simulink model "Experience"  (R2025b)
settings: Solver=ode1  StartTime=0.0  StopTime=inf  FixedStep=0.005  RelTol=1e-3  EnableMultiTasking=on
values from neighbouring files (symbols this model uses):
  A = model.a    [param_control.m]
  B = model.b    [param_control.m]
  C = model.c    [param_control.m]
  H = 1/ (C_cmd*((eye(4) - A + B*K)\B))    [param_control.m]
  K = place(A, B, z_p)    [param_control.m]
  L = place(A',C', z_po)'    [param_control.m]
  nx = 4    [ident_model.m]    (also in param_control.m)
undefined symbols (not defined in the file or in its folder): Ka
libraries: arduinolib x1
settings Model: SimulationMode=external  ExtModeTrigDuration=2  Creator=Alex  LastModifiedBy=victor
settings SolverCC: AlgebraicLoopSolver=TrustRegion
settings DataIOCC: SaveFormat=StructureWithTime  ReturnWorkspaceOutputs=off
settings OptimizationCC: DefaultUnderspecifiedDataType=single  ReuseModelBlockBuffer=off  PassReuseOutputArgsAs=Individual arguments  MaxStackSize=64  EfficientTunableParamExpr=on
settings DebuggingCC: ParameterPrecisionLossMsg=none  ParameterTunabilityLossMsg=error  UnconnectedInputMsg=warning  UnconnectedOutputMsg=warning  UnconnectedLineMsg=warning  ArithmeticOperatorsInVariantConditions=warning
settings HardwareCC: ProdBitPerInt=16.0  ProdBitPerPointer=16.0  ProdBitPerSizeT=16.0  ProdBitPerPtrDiffT=16.0  ProdLargestAtomicFloat=None  ProdWordSize=8.0  ProdHWDeviceType=Atmel->AVR
settings ModelReferenceCC: EnableRefExpFcnMdlSchedulingChecks=on
settings SFSimCC: SimUseLocalCustomCode=off  MATLABDynamicMemAlloc=off  CustomCodeUndefinedFunction=UseInterfaceOnly
settings RTWCC: SystemTargetFile=ert.tlc  HardwareBoard=Arduino Mega 2560  TemplateMakefile=ert_default_tmf  RTWUseLocalCustomCode=off  Toolchain=Arduino AVR  BuildConfiguration=Faster Runs  IncludeHyperlinkInReport=on  GPUComputeCapability=3.5  DLArmComputeVersion=19.05  Description=Embedded Coder
settings CodeAppCC: ForceParamTrailComments=on  IgnoreCustomStorageClasses=off  OperatorAnnotations=on  SimulinkDataObjDesc=on  SFDataObjDesc=on  InsertBlockDesc=on
settings ERTTargetCC: ExtModeTransport=3.0  ExtModeStaticAlloc=on  ExtModeStaticAllocSize=1000.0  ExtModeMexFile=ext_xcp  ExtModeIntrfLevel=Level2 - Open  InlinedParameterPlacement=Hierarchical  DynamicArrayContainerType=coder::array  SupportContinuousTime=on  SupportVariableSizeSignals=on
settings SimscapeCC: SimscapeLogDecimation=1  SimscapeLogDataHistory=5000

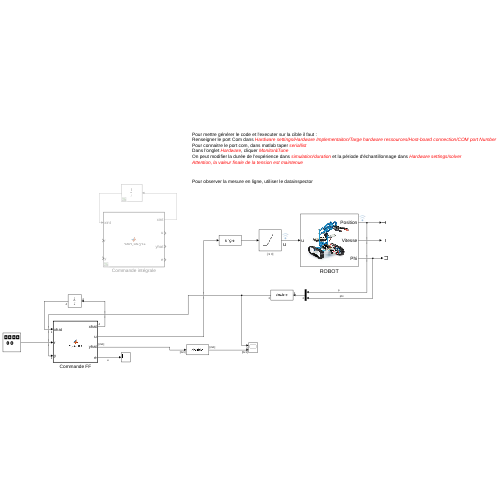
[thumbnail: Simulink's stored preview of the top-level diagram]
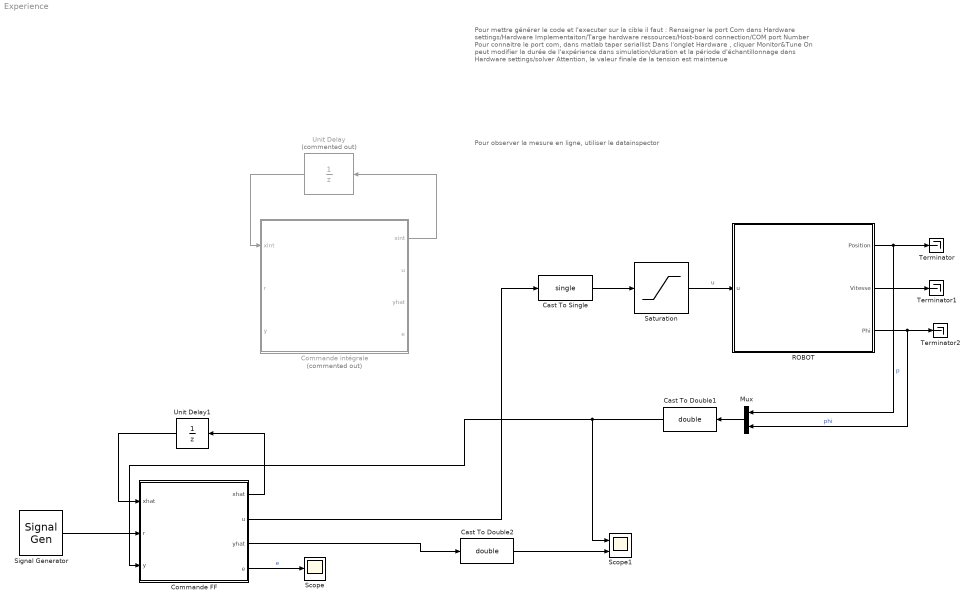
== system Experience ==
  note: Pour observer la mesure en ligne, utiliser le datainspector
  note: Pour mettre générer le code et l'executer sur la cible il faut :
      | Renseigner le port Com dans Hardware settings/Hardware Implementaiton/Targe hardware ressources/Host-board connection/COM port Number
      | Pour connaitre le port com, dans matlab taper seriallist
      | Dans l'onglet Hardware , cliquer Monitor&Tune
      | On peut modifier la durée de l'expérience dans simulation/duration et la période d'échantillonnage dans Hardware settings/solver
      | Attention, la valeur finale de la tension est maintenue
  Cast To Double1 : DataTypeConversion  OutDataTypeStr=double  SaturateOnIntegerOverflow=off  RndMeth=Floor
  Cast To Double2 : DataTypeConversion  OutDataTypeStr=double  SaturateOnIntegerOverflow=off  RndMeth=Floor
  Cast To Single : DataTypeConversion  OutDataTypeStr=single  SaturateOnIntegerOverflow=off  RndMeth=Floor
  Commande FF : MATLAB Function  TreatAsAtomicUnit=on
  Commande intégrale : MATLAB Function  Commented=on  TreatAsAtomicUnit=on
  Mux : Mux  Inputs=2
  ROBOT : Subsystem
      mask Display: image('robot_makeblock.jpg');
  Saturation : Saturate  UpperLimit=9  LowerLimit=-9
      settings: AttributesFormatString=[%<LowerLimit> %<UpperLimit>]
  Scope : Scope
  Scope1 : Scope  NumInputPorts=2
  Signal Generator : SignalGenerator  Amplitude=0  Frequency=.2
  Terminator : Terminator
  Terminator1 : Terminator
  Terminator2 : Terminator
  Unit Delay : UnitDelay  Commented=on  InitialCondition=zeros(nx+1,1)  SampleTime=-1  HasFrameUpgradeWarning=on
  Unit Delay1 : UnitDelay  InitialCondition=zeros(nx,1)  SampleTime=-1  HasFrameUpgradeWarning=on
  wires:
  Saturation/1 -> ROBOT/1(u)  "u"
  ROBOT/1(Position) -> Mux/1, Terminator/1  "p"
  ROBOT/2(Vitesse) -> Terminator1/1
  ROBOT/3(Phi) -> Mux/2, Terminator2/1  "phi"
  Commande intégrale/1(xint) -> Unit Delay/1
  Unit Delay/1 -> Commande intégrale/1("xint ")
  Unit Delay1/1 -> Commande FF/1("xhat ")
  Commande FF/1(xhat) -> Unit Delay1/1
  Cast To Single/1 -> Saturation/1
  Mux/1 -> Cast To Double1/1
  Signal Generator/1 -> Commande FF/2(r)
  Cast To Double1/1 -> Scope1/1, Commande FF/3(y)
  Commande FF/2(u) -> Cast To Single/1
  Commande FF/4(e) -> Scope/1  "e"
  Commande FF/3(yhat) -> Cast To Double2/1
  Cast To Double2/1 -> Scope1/2

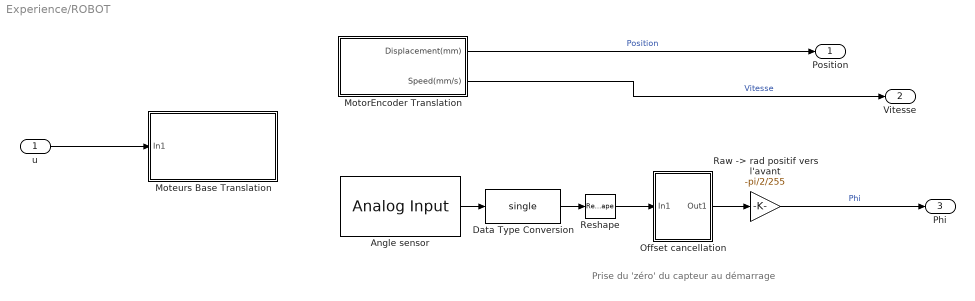
== system Experience/ROBOT ==
  note: Prise du 'zéro' du capteur au démarrage
  u : Inport
  Angle sensor : arduinolib/Analog Input  pinNumber=10  ReadResultsOnly=off  ConversionTriggerSource=Software  ExternalTriggerType=uint32(0)  OutputDataType=uint16  EnableConversionCompleteNotify=off  EnableOuputStatus=off  SampleTime=-1  blockPlatform=arduino
  Data Type Conversion : DataTypeConversion  OutDataTypeStr=single  SaturateOnIntegerOverflow=off  RndMeth=Floor
  Moteurs Base Translation : Subsystem
  MotorEncoder Translation : Subsystem  mask{pulsePerTurn=8, beltPitch=2.032, nTeeth=90, gearRatio=46}
      mask prompts: pulsePerTurn "Encoder resolution"; beltPitch "Belt Pitch"; nTeeth "Number of teeth"; gearRatio "Gear ratio"
  Offset cancellation : Subsystem
  "Raw -> rad positif vers l'avant" : Gain  Gain=-pi/2/255
  Reshape : Reshape  OutputDimensions=1
  Position : Outport
  Vitesse : Outport  Port=2
  Phi : Outport  Port=3
  wires:
  Angle sensor/1 -> Data Type Conversion/1
  Data Type Conversion/1 -> Reshape/1
  u/1 -> Moteurs Base Translation/1(In1)
  Offset cancellation/1(Out1) -> "Raw -> rad positif vers l'avant"/1
  "Raw -> rad positif vers l'avant"/1 -> Phi/1  "Phi"
  MotorEncoder Translation/1(Displacement(mm)) -> Position/1  "Position"
  Reshape/1 -> Offset cancellation/1(In1)
  MotorEncoder Translation/2(Speed(mm/s)) -> Vitesse/1  "Vitesse"

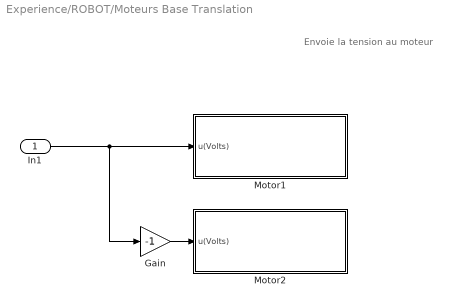
== system Experience/ROBOT/Moteurs Base Translation ==
  note: Envoie la tension au moteur
  In1 : Inport
  Gain : Gain  Gain=-1
  Motor1 : Subsystem  mask{Vmax=12}
      mask prompts: Vmax "Power supply Voltage"
  Motor2 : Subsystem  mask{Vmax=12}
      mask prompts: Vmax "Power supply Voltage"
  wires:
  Gain/1 -> Motor2/1(u(Volts))
  In1/1 -> Gain/1, Motor1/1(u(Volts))

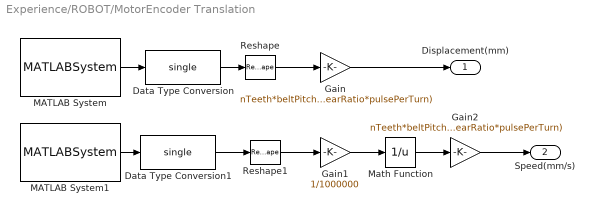
== system Experience/ROBOT/MotorEncoder Translation ==
  Data Type Conversion : DataTypeConversion  OutDataTypeStr=single  SaturateOnIntegerOverflow=off  RndMeth=Floor
  Data Type Conversion1 : DataTypeConversion  OutDataTypeStr=single  SaturateOnIntegerOverflow=off  RndMeth=Floor
  Gain : Gain  Gain=nTeeth*beltPitch/(gearRatio*pulsePerTurn)  OutDataTypeStr=single
      settings: AttributesFormatString=%<Gain>
  Gain1 : Gain  Gain=1/1000000
  Gain2 : Gain  Gain=nTeeth*beltPitch/(gearRatio*pulsePerTurn)  OutDataTypeStr=single
      settings: AttributesFormatString=%<Gain>
  MATLAB System : MATLABSystem  System=Enc1Read  SampleTime=-1
      mask Type: Enc1Read
  MATLAB System1 : MATLABSystem  System=Enc1Period  SampleTime=-1
      mask Type: Enc1Period
  Math Function : Math  Operator=reciprocal  SignedPower=on  OutputSignalType=real  OutDataTypeStr=single  SaturateOnIntegerOverflow=off
  Reshape : Reshape  OutputDimensions=1
  Reshape1 : Reshape  OutputDimensions=1
  Displacement(mm) : Outport  VectorParamsAs1DForOutWhenUnconnected=off
  Speed(mm/s) : Outport  Port=2  VectorParamsAs1DForOutWhenUnconnected=off
  wires:
  MATLAB System/1 -> Data Type Conversion/1
  Data Type Conversion/1 -> Reshape/1
  Gain1/1 -> Math Function/1
  Data Type Conversion1/1 -> Reshape1/1
  MATLAB System1/1 -> Data Type Conversion1/1
  Math Function/1 -> Gain2/1
  Gain2/1 -> Speed(mm/s)/1
  Gain/1 -> Displacement(mm)/1
  Reshape/1 -> Gain/1
  Reshape1/1 -> Gain1/1

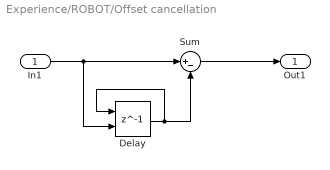
== system Experience/ROBOT/Offset cancellation ==
  In1 : Inport
  Delay : Delay  DelayLength=1  InitialConditionSource=Input port
      settings: InputPortMap=u0,p4
  Sum : Sum  Inputs=|+-
  Out1 : Outport  VectorParamsAs1DForOutWhenUnconnected=off
  wires:
  In1/1 -> Sum/1, Delay/2
  Delay/1 -> Sum/2, Delay/1
  Sum/1 -> Out1/1

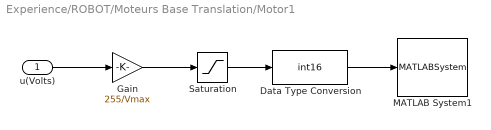
== system Experience/ROBOT/Moteurs Base Translation/Motor1 ==
  u(Volts) : Inport
  Data Type Conversion : DataTypeConversion  OutDataTypeStr=int16  SaturateOnIntegerOverflow=off  RndMeth=Floor
  Gain : Gain  Gain=255/Vmax
      settings: AttributesFormatString=%<Gain>
  MATLAB System1 : MATLABSystem  System=DCMotor1Set
      mask Type: DCMotor1Set
  Saturation : Saturate  UpperLimit=255  LowerLimit=-255
  wires:
  Gain/1 -> Saturation/1
  u(Volts)/1 -> Gain/1
  Data Type Conversion/1 -> MATLAB System1/1
  Saturation/1 -> Data Type Conversion/1

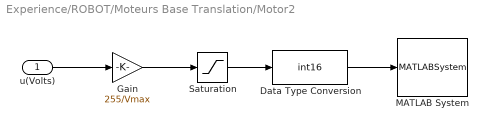
== system Experience/ROBOT/Moteurs Base Translation/Motor2 ==
  u(Volts) : Inport
  Data Type Conversion : DataTypeConversion  OutDataTypeStr=int16  SaturateOnIntegerOverflow=off  RndMeth=Floor
  Gain : Gain  Gain=255/Vmax
      settings: AttributesFormatString=%<Gain>
  MATLAB System : MATLABSystem  System=DCMotor2Set
      mask Type: DCMotor2Set
  Saturation : Saturate  UpperLimit=255  LowerLimit=-255
  wires:
  Saturation/1 -> Data Type Conversion/1
  Data Type Conversion/1 -> MATLAB System/1
  u(Volts)/1 -> Gain/1
  Gain/1 -> Saturation/1

== matlab function Experience/Commande FF ==
  data: xhat output; xhat input; r input; u output; y input; L parameter; C parameter; B parameter; A parameter; K parameter; yhat output; e output; H parameter
function [xhat,u,yhat,e] = ControlFF(xhat,r,y,L, C, B, A, K, H)

z = y(1);
e = r-z;
u = -K*xhat+H*r; 

yhat = C*xhat;
xhat = A*xhat+B*u+L*(y-yhat);

== matlab function Experience/Commande intégrale ==
  data: xint output; xint input; r input; u output; y input; Ka parameter; L parameter; C parameter; B parameter; A parameter; yhat output; e output
function [xint,u,yhat,e] = Control_Integrale(xint,r,y,Ka, L, C, B, A)

z = y(1);
xhat = xint(1:4);
eta = xint(5);
e = r-z;
u = -Ka*xint;
 
yhat = C*xhat;
xhat = A*xhat+B*u+L*(y-yhat);
eta = eta+e;
%eta = eta+e+Kb*(u_sat-u);
xint = [xhat;eta];
